simulink model "Part1_FIXED"  (R2024b)
settings: Solver=VariableStepAuto  StartTime=0.0  StopTime=T_SIM  RelTol=1e-3
values from neighbouring files (symbols this model uses):
  T_s = (sim_output.tout(end)-sim_output.tout(1))/(length(sim_output.tout)-1)    [P1_save_data.m]
undefined symbols (not defined in the file or in its folder): d, r, R, Ta, Tc, w, w_max, X, Y
libraries: robotlib x6, sharedtransform x1
settings Model: Creator=llp  LastModifiedBy=llp

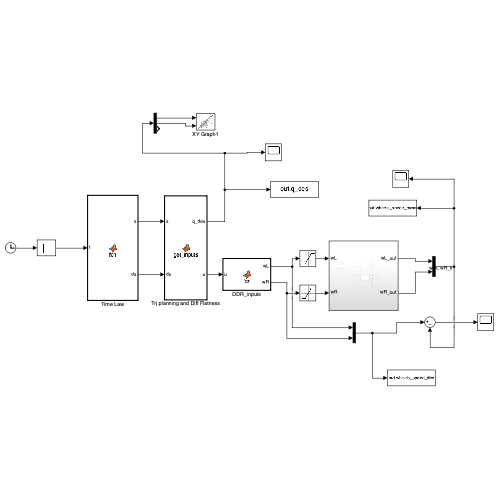
[thumbnail: Simulink's stored preview of the top-level diagram]
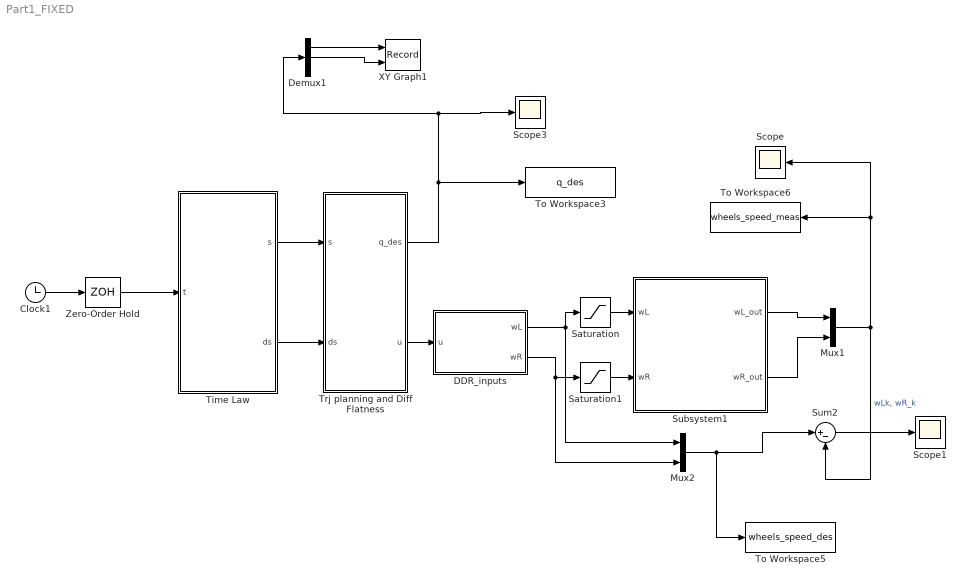
== system Part1_FIXED ==
  Clock1 : Clock
      settings: Decimation=1/T_s
  DDR_inputs : MATLAB Function  TreatAsAtomicUnit=on
  Demux1 : Demux  Outputs=3
  Mux1 : Mux  Inputs=2
  Mux2 : Mux  Inputs=2
  Saturation : Saturate  UpperLimit=w_max  LowerLimit=-w_max
  Saturation1 : Saturate  UpperLimit=w_max  LowerLimit=-w_max
  Scope : Scope
  Scope1 : Scope
  Scope3 : Scope
  Subsystem1 : Subsystem
  Sum2 : Sum  Inputs=|+-
  Time Law : MATLAB Function  TreatAsAtomicUnit=on
  To Workspace3 : ToWorkspace  VariableName=q_des  SaveFormat=Structure With Time  SampleTime=-1
  To Workspace5 : ToWorkspace  VariableName=wheels_speed_des  SaveFormat=Structure With Time  SampleTime=-1
  To Workspace6 : ToWorkspace  VariableName=wheels_speed_meas  SaveFormat=Structure With Time  SampleTime=-1
  Trj planning and Diff Flatness : MATLAB Function  TreatAsAtomicUnit=on
  XY Graph1 : Record  FileSettingsInternal="{\"entries\":[{\"content\":{\"excelSettings\":{\"content\":{},\"type\":\"Streamout.ExcelSettings\"}},\"type\":\"Streamout.FileSettingStorage\",\"uuid\":\"\"}],\"packageUris\":[\"http:\\/\\/schema.mathworks.com\\/mf0\\/streamout_blocks\\/R2020a\"],\"version\":\"1.0\"}"  Layout=[1 1]  SignalsInternal="{\"entries\":[{\"content\":{\"signals\":[{\"content\":{\"blockPath\":[],\"dimensions\":[1,1],\"domain\":\"\",\"lineColor\":\"#a2142f\",\"plots\":[ 1 ],\"port\":1,\"sid\":[\"\"],\"signalID\":1,\"signalName\":\"Demux1:1\"},\"type\":\"RecordBlkView.Signal\",\"uuid\":\"\"},{\"content\":{\"blockPath\":[],\"dimensions\":[1,1],\"domain\":\"\",\"lineColor\":\"#139fff\",\"plots\":[ 1 ],\"port\":2,\"sid\":[\"\"],\"signalID\":2,\"signalName\":\"Demux1:2\"},\"type\":\"RecordBlkView.Signal\",\"uuid\":\"\"}]},\"type\":\"RecordBlkView.InputSignals\",\"uuid\":\"\"}],\"packageUris\":[\"http:\\/\\/schema.mathworks.com\\/mf0\\/streamout_blocks\\/R2020a\"],\"version\":\"1.0\"}"  VisualizationBindings="{\"xyplotplugin\":{\"info\":[{\"series\":[{\"bindingParametersList\":[{\"parameter\":\"X-Axis\",\"signalID\":1,\"signalName\":\"Demux1:1\"},{\"parameter\":\"Y-Axis\",\"signalID\":2,\"signalName\":\"Demux1:2\"}],\"seriesID\":0}],\"subplotID\":1}]}}"  CompatibilityTag=XY
  Zero-Order Hold : ZeroOrderHold  SampleTime=T_s
  wires:
  Zero-Order Hold/1 -> Time Law/1(t)
  Saturation1/1 -> Subsystem1/2(wR)
  DDR_inputs/2(wR) -> Mux2/2, Saturation1/1
  Saturation/1 -> Subsystem1/1(wL)
  Mux1/1 -> Sum2/2, Scope/1, To Workspace6/1  "wLk, wR_k"
  Trj planning and Diff Flatness/1(q_des) -> To Workspace3/1, Scope3/1, Demux1/1
  Trj planning and Diff Flatness/2(u) -> DDR_inputs/1(u)
  Subsystem1/1(wL_out) -> Mux1/1
  Subsystem1/2(wR_out) -> Mux1/2
  Demux1/2 -> XY Graph1/2
  Time Law/1(s) -> Trj planning and Diff Flatness/1(s)
  DDR_inputs/1(wL) -> Saturation/1, Mux2/1
  Clock1/1 -> Zero-Order Hold/1
  Demux1/1 -> XY Graph1/1
  Time Law/2(ds) -> Trj planning and Diff Flatness/2(ds)
  Mux2/1 -> To Workspace5/1, Sum2/1
  Sum2/1 -> Scope1/1

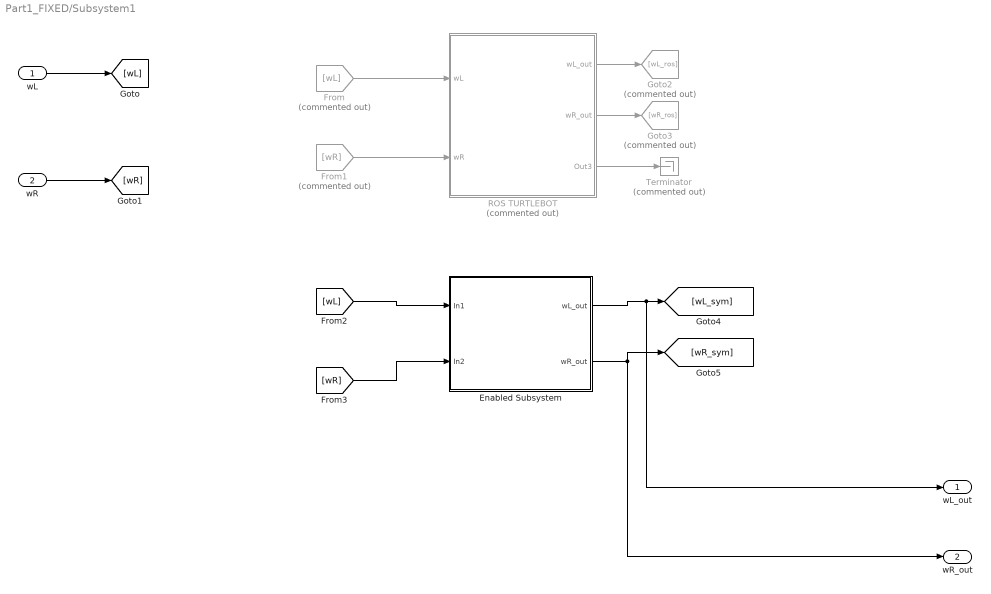
== system Part1_FIXED/Subsystem1 ==
  wL : Inport
  wR : Inport  Port=2
  Enabled Subsystem : Subsystem  TreatAsAtomicUnit=on
  From : From  Commented=on  GotoTag=wL
  From1 : From  Commented=on  GotoTag=wR
  Goto2 : Goto  Commented=on  GotoTag=wL_ros
  Goto3 : Goto  Commented=on  GotoTag=wR_ros
  ROS TURTLEBOT : Subsystem  Commented=on
  Terminator : Terminator  Commented=on
  wL_out : Outport
  wR_out : Outport  Port=2
  wires:
  ROS TURTLEBOT/3(Out3) -> Terminator/1
  wL/1 -> [wL]
  wR/1 -> [wR]
  ROS TURTLEBOT/1(wL_out) -> Goto2/1
  ROS TURTLEBOT/2(wR_out) -> Goto3/1
  From/1 -> ROS TURTLEBOT/1(wL)
  From1/1 -> ROS TURTLEBOT/2(wR)
  [wL] -> Enabled Subsystem/1(In1)
  [wR] -> Enabled Subsystem/2(In2)
  Enabled Subsystem/1(wL_out) -> wL_out/1, [wL_sym]
  Enabled Subsystem/2(wR_out) -> wR_out/1, [wR_sym]

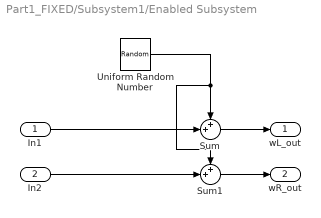
== system Part1_FIXED/Subsystem1/Enabled Subsystem ==
  In1 : Inport
  In2 : Inport  Port=2
  Sum : Sum  Inputs=++|
  Sum1 : Sum  Inputs=++|
  Uniform Random Number : UniformRandomNumber  SampleTime=T_s
  wL_out : Outport
  wR_out : Outport  Port=2
  wires:
  In1/1 -> Sum/2
  Sum/1 -> wL_out/1
  Uniform Random Number/1 -> Sum1/1, Sum/1
  In2/1 -> Sum1/2
  Sum1/1 -> wR_out/1

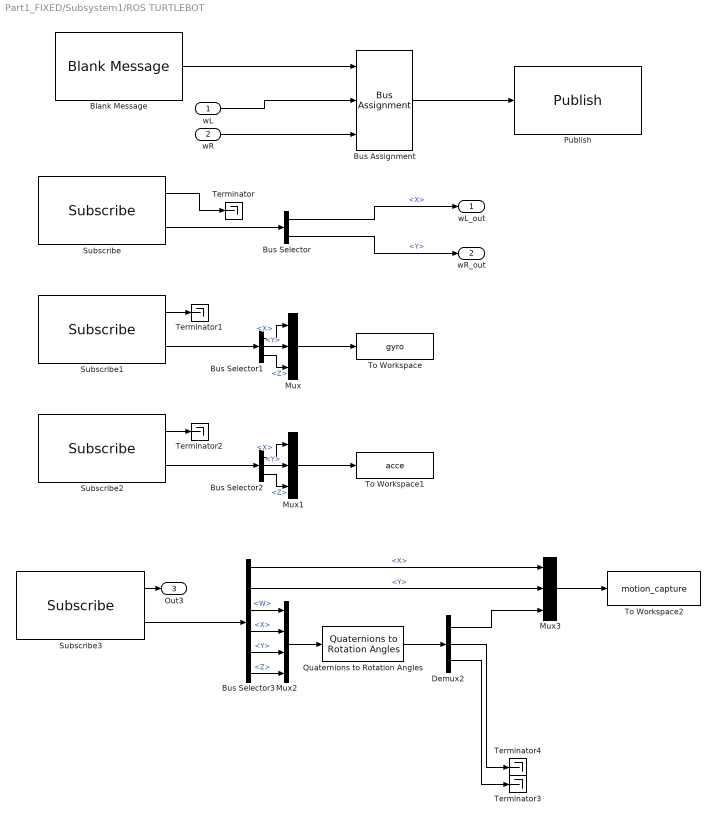
== system Part1_FIXED/Subsystem1/ROS TURTLEBOT ==
  wL : Inport
  wR : Inport  Port=2
  Blank Message : robotlib/Blank Message  messageClass=Message  entityType=geometry_msgs/Vector3  messageType=geometry_msgs/Vector3  SampleTime=T_s  legacyBusStruct=off
  Bus Assignment : BusAssignment  AssignedSignals=X,Y
  Bus Selector : BusSelector  OutputSignals=X,Y
  Bus Selector1 : BusSelector  OutputSignals=X,Y,Z
  Bus Selector2 : BusSelector  OutputSignals=X,Y,Z
  Bus Selector3 : BusSelector  OutputSignals=Pose.Pose.Position.X,Pose.Pose.Position.Y,Pose.Pose.Orientation.W,Pose.Pose.Orientation.X,Pose.Pose.Orientation.Y,Pose.Pose.Orientation.Z
  Demux2 : Demux  Outputs=3
  Mux : Mux  Inputs=3
  Mux1 : Mux  Inputs=3
  Mux2 : Mux
  Mux3 : Mux  Inputs=3
  Publish : robotlib/Publish  topicSource=Select from ROS network  topic=/turtlebot_01/cmd_wheels  messageType=geometry_msgs/Vector3  legacyBusStruct=off  messageQueueLength=1
  Quaternions to Rotation Angles : sharedtransform/Quaternions to Rotation Angles  rotationOrder=ZYX  aMode=aMode
  Subscribe : robotlib/Subscribe  topicSource=Select from ROS network  topic=/turtlebot_01/wheelSpeeds  messageType=geometry_msgs/Vector3  SampleTime=T_s  legacyBusStruct=off  messageQueueLength=1
  Subscribe1 : robotlib/Subscribe  topicSource=Select from ROS network  topic=/turtlebot_01/gyroscope  messageType=geometry_msgs/Vector3  SampleTime=T_s  legacyBusStruct=off  messageQueueLength=1
  Subscribe2 : robotlib/Subscribe  topicSource=Select from ROS network  topic=/turtlebot_01/accelerometer  messageType=geometry_msgs/Vector3  SampleTime=T_s  legacyBusStruct=off  messageQueueLength=1
  Subscribe3 : robotlib/Subscribe  topicSource=Select from ROS network  topic=/turtlebot_01/odom  messageType=nav_msgs/Odometry  SampleTime=T_s  legacyBusStruct=off  messageQueueLength=1
      settings: LibrarySourceBlock=roslib/ROS/Subscribe
  Terminator{,1..4} (5 alike) : Terminator
  To Workspace : ToWorkspace  VariableName=gyro  SaveFormat=Structure With Time  SampleTime=-1
  To Workspace1 : ToWorkspace  VariableName=acce  SaveFormat=Structure With Time  SampleTime=-1
  To Workspace2 : ToWorkspace  VariableName=motion_capture  SaveFormat=Structure With Time  SampleTime=-1
  wL_out : Outport
  wR_out : Outport  Port=2
  Out3 : Outport  Port=3
  wires:
  Subscribe3/1 -> Out3/1
  Bus Selector3/3 -> Mux2/1  "<W>"
  Quaternions to Rotation Angles/1 -> Demux2/1
  Mux1/1 -> To Workspace1/1
  Mux2/1 -> Quaternions to Rotation Angles/1
  Subscribe/1 -> Terminator/1
  Bus Assignment/1 -> Publish/1
  Subscribe3/2 -> Bus Selector3/1
  Bus Selector3/6 -> Mux2/4  "<Z>"
  Bus Selector2/3 -> Mux1/3  "<Z>"
  Subscribe2/1 -> Terminator2/1
  Bus Selector1/1 -> Mux/1  "<X>"
  Mux/1 -> To Workspace/1
  Subscribe1/1 -> Terminator1/1
  Demux2/1 -> Mux3/3
  Subscribe/2 -> Bus Selector/1
  Demux2/2 -> Terminator4/1
  Bus Selector3/5 -> Mux2/3  "<Y>"
  Bus Selector3/2 -> Mux3/2  "<Y>"
  Bus Selector1/3 -> Mux/3  "<Z>"
  Subscribe2/2 -> Bus Selector2/1
  Bus Selector3/1 -> Mux3/1  "<X>"
  Blank Message/1 -> Bus Assignment/1
  Bus Selector2/1 -> Mux1/1  "<X>"
  Bus Selector1/2 -> Mux/2  "<Y>"
  Bus Selector/1 -> wL_out/1  "<X>"
  wL/1 -> Bus Assignment/2
  Mux3/1 -> To Workspace2/1
  Subscribe1/2 -> Bus Selector1/1
  wR/1 -> Bus Assignment/3
  Demux2/3 -> Terminator3/1
  Bus Selector3/4 -> Mux2/2  "<X>"
  Bus Selector/2 -> wR_out/1  "<Y>"
  Bus Selector2/2 -> Mux1/2  "<Y>"

== matlab function Part1_FIXED/Time Law ==
  data: t input; s output; ds output; Ta parameter; Tc parameter
function [s, ds] = fcn(t, Ta, Tc)
          
    vc = 1/(Ta+Tc);
    a = vc/Ta;
   
    if t < Ta
        s_dot = a*t;
        s = 0.5*a*t^2;
    
    elseif t < (Ta+Tc)
        s_dot = vc;
        s = 0.5*a*Ta^2 + vc*(t - Ta);
    
    elseif t < (2*Ta+Tc)
        s_dot = vc - a*(t - Ta - Tc);
        s = 0.5*a*Ta^2 + vc*Tc + vc*(t - Ta - Tc) ...
            - 0.5*a*(t - Ta - Tc)^2;
    else
        s_dot = 0;
        s = 1;
    end

    ds = s_dot;
    
end

== matlab function Part1_FIXED/Trj planning and Diff Flatness ==
  data: q_des output; s input; u output; ds input; R parameter; w parameter
function [q_des, u] = get_inputs(s, ds, R, w)

    % function [x_s, y_s, x_s_dot, y_s_dot, x_s_ddot, y_s_ddot] = gen_eight_shape_trajectory(R, w, s)
   
    x_s = R*sin(2*w*s);
    y_s = R*sin(w*s);
    
    % computes derivatives analytically

    x_s_dot = 2*R*w*cos(2*w*s);
    y_s_dot = R*w*cos(w*s);
    
    x_s_ddot = -4*R*w^2*sin(2*w*s);
    y_s_ddot = -R*w^2*sin(w*s);


    % function [q, u] = flat_to_kinematic_cartesian(x, y, x_dot, y_dot, x_ddot, y_ddot)

    theta = atan2(y_s_dot, x_s_dot);
    
    q_des = [x_s; y_s; theta];
   
    v_tilde = sqrt(x_s_dot^2 + y_s_dot^2);
    omega_tilde = (x_s_dot * y_s_ddot - y_s_dot * x_s_ddot) / (x_s_dot^2 + y_s_dot^2);
    
    % Convert into real Inputs
    v = v_tilde * ds;
    omega = omega_tilde * ds;
    
    u = [v; omega];
end

== matlab function Part1_FIXED/DDR_inputs ==
  data: u input; wL output; wR output; r parameter; d parameter
function [wL, wR] = fcn(u,r, d)

    v = u(1);
    omega = u(2);

    wL = v/r - (d*omega)/(2*r);
    wR = v/r + (d*omega)/(2*r);

end
